simulink model "kf_test"  (R2018b)
settings: Solver=ode2  StartTime=0  StopTime=200  FixedStep=0.002  RelTol=1e-3  EnableMultiTasking=on
model workspace (MAT data in the model file):
  m = 1000
undefined symbols (not defined in the file or in its folder): t_EstimateLoc1_s, t_EstimateLoc2_s, TUMVehicleState
libraries: simulink x6
settings Model: DataDictionary=kf_test.sldd  PauseTimes=42.1  Creator=wischnewski  LastModifiedBy=ge34qer
settings DataIOCC: ExternalInput=input  LoadExternalInput=on  SaveFormat=Structure
settings OptimizationCC: LifeSpan=inf
settings DebuggingCC: MultiTaskRateTransMsg=warning
settings SFSimCC: SimUseLocalCustomCode=off
settings RTWCC: RTWUseLocalCustomCode=off
settings CodeAppCC: StateflowObjectComments=on

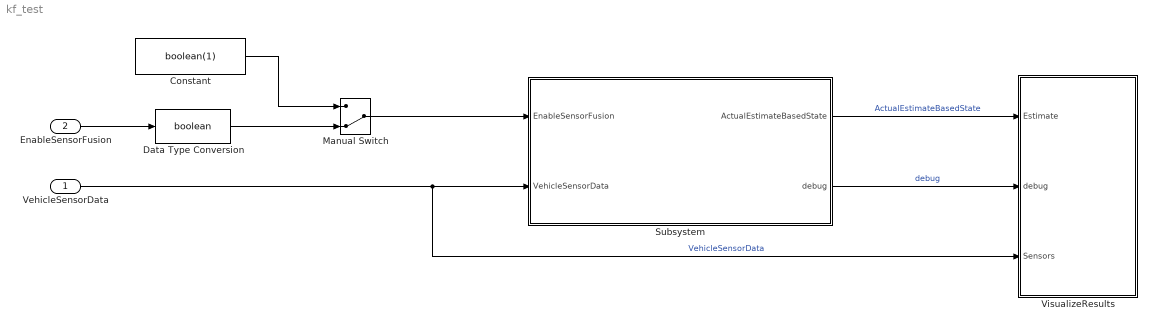
== system kf_test ==
  VehicleSensorData : Inport  OutDataTypeStr=Bus: VehicleSensorData
  EnableSensorFusion : Inport  Port=2  OutDataTypeStr=uint16
  Constant : Constant  Value=boolean(1)
  Data Type Conversion : DataTypeConversion  OutDataTypeStr=boolean
  Manual Switch : ManualSwitch  CurrentSetting=0
  Subsystem : Subsystem
  VisualizeResults : Subsystem
  wires:
  VehicleSensorData/1 -> VisualizeResults/3(Sensors), Subsystem/2(VehicleSensorData)  "VehicleSensorData"
  Subsystem/1(ActualEstimateBasedState) -> VisualizeResults/1(Estimate)  "ActualEstimateBasedState"
  Subsystem/2(debug) -> VisualizeResults/2(debug)  "debug"
  EnableSensorFusion/1 -> Data Type Conversion/1
  Constant/1 -> Manual Switch/1
  Data Type Conversion/1 -> Manual Switch/2
  Manual Switch/1 -> Subsystem/1(EnableSensorFusion)

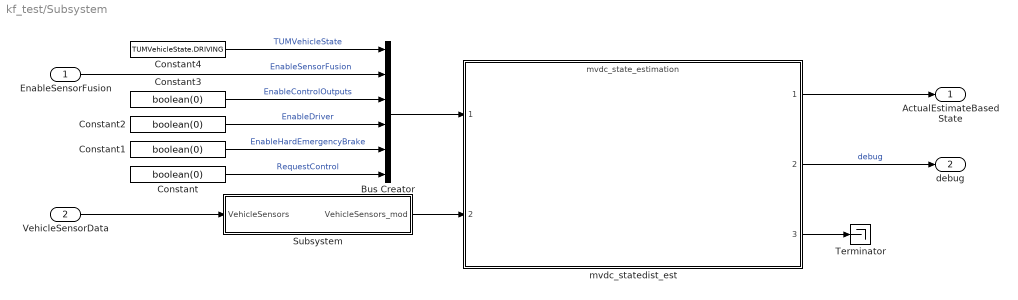
== system kf_test/Subsystem ==
  EnableSensorFusion : Inport
  VehicleSensorData : Inport  Port=2
  Bus Creator : BusCreator  Inputs=6
  Constant{,1..3} (4 alike) : Constant  Value=boolean(0)
  Constant4 : Constant  Value=TUMVehicleState.DRIVING
  Subsystem : Subsystem
  Terminator : Terminator
  mvdc_statedist_est : ModelReference  ModelNameDialog=mvdc_state_estimation  SimulationMode=Normal  ModelReferenceVersion=1.939
  ActualEstimateBasedState : Outport
  debug : Outport  Port=2
  wires:
  mvdc_statedist_est/1 -> ActualEstimateBasedState/1
  mvdc_statedist_est/2 -> debug/1  "debug"
  VehicleSensorData/1 -> Subsystem/1(VehicleSensors)
  Subsystem/1(VehicleSensors_mod) -> mvdc_statedist_est/2
  mvdc_statedist_est/3 -> Terminator/1
  Bus Creator/1 -> mvdc_statedist_est/1
  Constant/1 -> Bus Creator/6  "RequestControl"
  Constant1/1 -> Bus Creator/5  "EnableHardEmergencyBrake"
  Constant2/1 -> Bus Creator/4  "EnableDriver"
  Constant3/1 -> Bus Creator/3  "EnableControlOutputs"
  Constant4/1 -> Bus Creator/1  "TUMVehicleState"
  EnableSensorFusion/1 -> Bus Creator/2  "EnableSensorFusion"

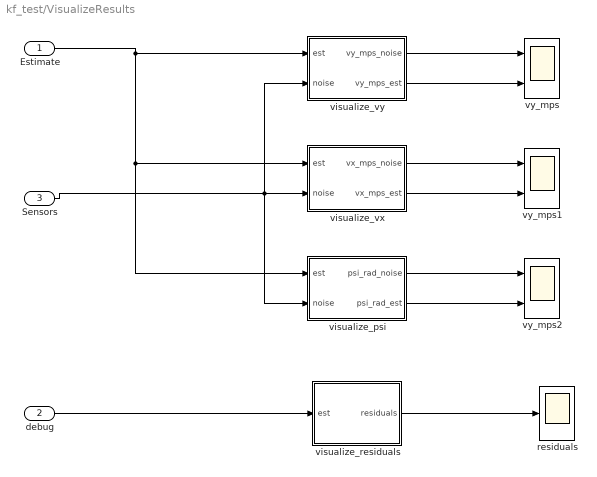
== system kf_test/VisualizeResults ==
  Estimate : Inport
  debug : Inport  Port=2
  Sensors : Inport  Port=3
  residuals : Scope
  visualize_psi : Subsystem
  visualize_residuals : Subsystem
  visualize_vx : Subsystem
  visualize_vy : Subsystem
  vy_mps : Scope  NumInputPorts=2
  vy_mps1 : Scope  NumInputPorts=2
  vy_mps2 : Scope  NumInputPorts=2
  wires:
  visualize_residuals/1(residuals) -> residuals/1
  Estimate/1 -> visualize_psi/1(est), visualize_vx/1(est), visualize_vy/1(est)
  Sensors/1 -> visualize_psi/2(noise), visualize_vy/2(noise), visualize_vx/2(noise)
  debug/1 -> visualize_residuals/1(est)
  visualize_vy/1(vy_mps_noise) -> vy_mps/1
  visualize_vy/2(vy_mps_est) -> vy_mps/2
  visualize_vx/1(vx_mps_noise) -> vy_mps1/1
  visualize_vx/2(vx_mps_est) -> vy_mps1/2
  visualize_psi/1(psi_rad_noise) -> vy_mps2/1
  visualize_psi/2(psi_rad_est) -> vy_mps2/2

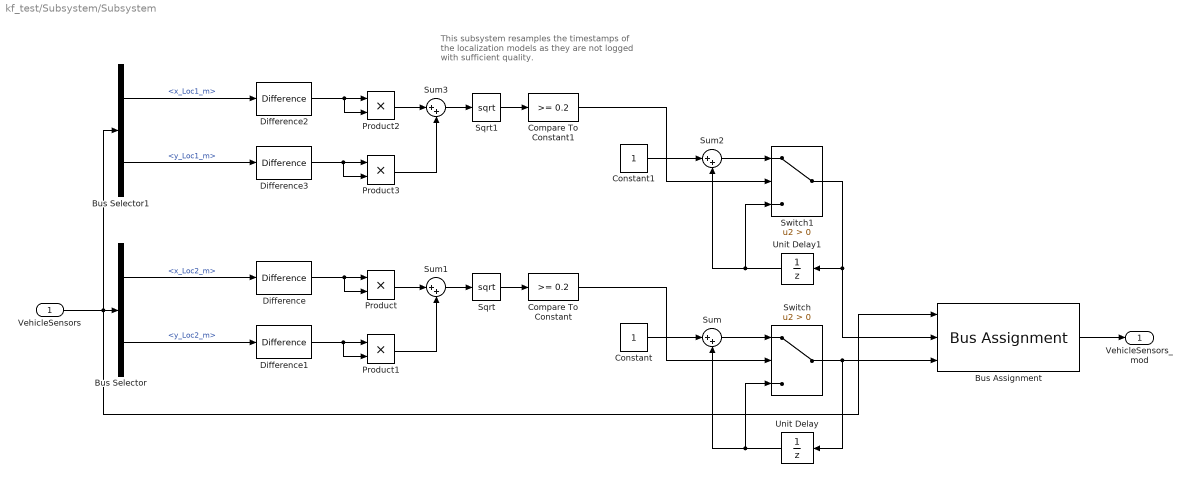
== system kf_test/Subsystem/Subsystem ==
  note: This subsystem resamples the timestamps
      | of the localization models as they are not
      | logged with sufficient quality.
  VehicleSensors : Inport
  Bus Assignment : BusAssignment  AssignedSignals=t_EstimateLoc1_s,t_EstimateLoc2_s
  Bus Selector : BusSelector  OutputSignals=x_Loc2_m,y_Loc2_m
  Bus Selector1 : BusSelector  OutputSignals=x_Loc1_m,y_Loc1_m
  Compare To Constant : simulink/Logic and Bit Operations/Compare To Constant  relop=>=  const=0.2  OutDataTypeStr=boolean
  Compare To Constant1 : simulink/Logic and Bit Operations/Compare To Constant  relop=>=  const=0.2  OutDataTypeStr=boolean
  Constant : Constant
  Constant1 : Constant
  Difference{,1..3} (4 alike) : simulink/Discrete/Difference  ICPrevInput=0.0  OutMin=[]  OutMax=[]  OutDataType=fixdt(1, 16)  OutScaling=2^-10  DoSatur=off
  Product{,1..3} (4 alike) : Product
  Sqrt : Sqrt  SaturateOnIntegerOverflow=on
  Sqrt1 : Sqrt  SaturateOnIntegerOverflow=on
  Sum{,1..3} (4 alike) : Sum  Inputs=|++
  Switch : Switch  Criteria=u2 > Threshold
  Switch1 : Switch  Criteria=u2 > Threshold
  Unit Delay : UnitDelay  SampleTime=-1
  Unit Delay1 : UnitDelay  SampleTime=-1
  VehicleSensors_mod : Outport
  wires:
  Bus Selector/2 -> Difference1/1  "<y_Loc2_m>"
  Unit Delay/1 -> Sum/2, Switch/3
  Difference1/1 -> Product1/2, Product1/1
  Sqrt/1 -> Compare To Constant/1
  Product/1 -> Sum1/1
  Switch/1 -> Unit Delay/1, Bus Assignment/3
  Bus Assignment/1 -> VehicleSensors_mod/1
  Constant/1 -> Sum/1
  Product1/1 -> Sum1/2
  Sum1/1 -> Sqrt/1
  VehicleSensors/1 -> Bus Assignment/1, Bus Selector1/1, Bus Selector/1
  Sum/1 -> Switch/1
  Difference/1 -> Product/2, Product/1
  Bus Selector/1 -> Difference/1  "<x_Loc2_m>"
  Compare To Constant/1 -> Switch/2
  Compare To Constant1/1 -> Switch1/2
  Sqrt1/1 -> Compare To Constant1/1
  Bus Selector1/1 -> Difference2/1  "<x_Loc1_m>"
  Unit Delay1/1 -> Sum2/2, Switch1/3
  Product2/1 -> Sum3/1
  Sum2/1 -> Switch1/1
  Difference3/1 -> Product3/2, Product3/1
  Difference2/1 -> Product2/2, Product2/1
  Switch1/1 -> Bus Assignment/2, Unit Delay1/1
  Bus Selector1/2 -> Difference3/1  "<y_Loc1_m>"
  Constant1/1 -> Sum2/1
  Sum3/1 -> Sqrt1/1
  Product3/1 -> Sum3/2

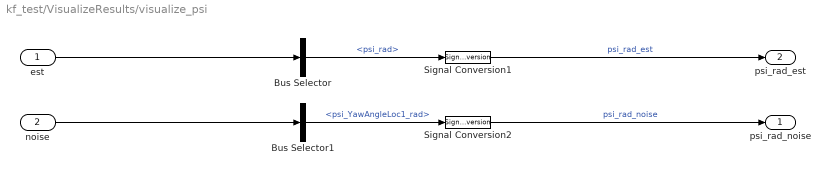
== system kf_test/VisualizeResults/visualize_psi ==
  est : Inport
  noise : Inport  Port=2
  Bus Selector : BusSelector  OutputSignals=Pos.psi_rad
  Bus Selector1 : BusSelector  OutputSignals=psi_YawAngleLoc1_rad
  Signal Conversion1 : SignalConversion  OverrideOpt=off
  Signal Conversion2 : SignalConversion  OverrideOpt=off
  psi_rad_noise : Outport
  psi_rad_est : Outport  Port=2
  wires:
  noise/1 -> Bus Selector1/1
  est/1 -> Bus Selector/1
  Signal Conversion1/1 -> psi_rad_est/1  "psi_rad_est"
  Signal Conversion2/1 -> psi_rad_noise/1  "psi_rad_noise"
  Bus Selector/1 -> Signal Conversion1/1  "<psi_rad>"
  Bus Selector1/1 -> Signal Conversion2/1  "<psi_YawAngleLoc1_rad>"

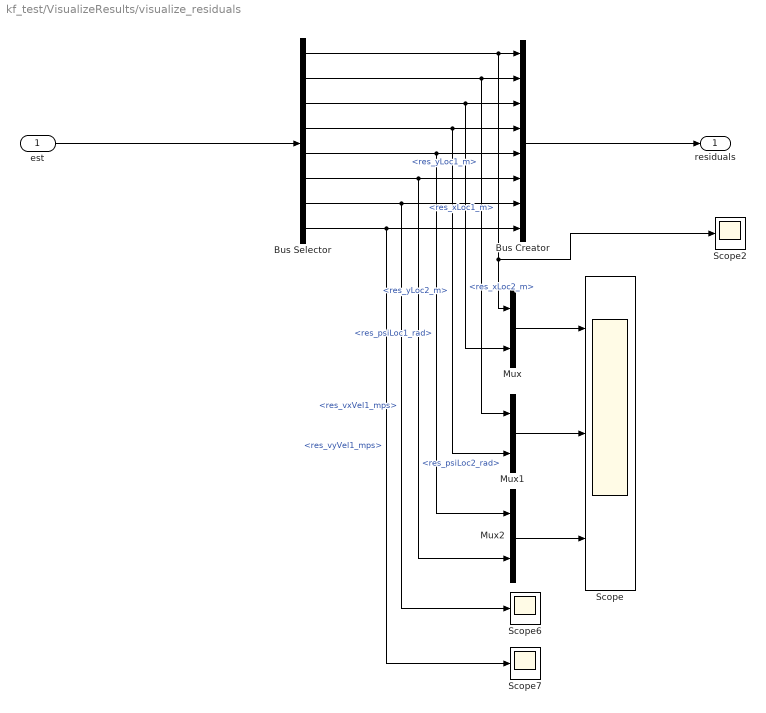
== system kf_test/VisualizeResults/visualize_residuals ==
  est : Inport
  Bus Creator : BusCreator  Inputs=8
  Bus Selector : BusSelector  OutputSignals=Residuals.res_xLoc1_m,Residuals.res_yLoc1_m,Residuals.res_xLoc2_m,Residuals.res_yLoc2_m,Residuals.res_psiLoc1_rad,Residuals.res_psiLoc2_rad,Residuals.res_vxVel1_mps,Residuals.res_vyVel1_mps
  Mux : Mux  Inputs=2
  Mux1 : Mux  Inputs=2
  Mux2 : Mux  Inputs=2
  Scope : Scope  NumInputPorts=3
  Scope2 : Scope
  Scope6 : Scope
  Scope7 : Scope
  residuals : Outport
  wires:
  Bus Selector/1 -> Scope2/1, Mux/1, Bus Creator/1  "<res_xLoc1_m>"
  est/1 -> Bus Selector/1
  Bus Selector/2 -> Mux1/1, Bus Creator/2  "<res_yLoc1_m>"
  Bus Selector/3 -> Mux/2, Bus Creator/3  "<res_xLoc2_m>"
  Bus Selector/5 -> Mux2/1, Bus Creator/5  "<res_psiLoc1_rad>"
  Bus Selector/4 -> Mux1/2, Bus Creator/4  "<res_yLoc2_m>"
  Bus Selector/6 -> Mux2/2, Bus Creator/6  "<res_psiLoc2_rad>"
  Bus Selector/7 -> Scope6/1, Bus Creator/7  "<res_vxVel1_mps>"
  Bus Selector/8 -> Scope7/1, Bus Creator/8  "<res_vyVel1_mps>"
  Bus Creator/1 -> residuals/1
  Mux1/1 -> Scope/2
  Mux/1 -> Scope/1
  Mux2/1 -> Scope/3

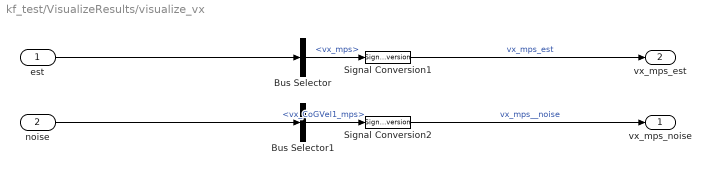
== system kf_test/VisualizeResults/visualize_vx ==
  est : Inport
  noise : Inport  Port=2
  Bus Selector : BusSelector  OutputSignals=vx_mps
  Bus Selector1 : BusSelector  OutputSignals=vx_CoGVel1_mps
  Signal Conversion1 : SignalConversion  OverrideOpt=off
  Signal Conversion2 : SignalConversion  OverrideOpt=off
  vx_mps_noise : Outport
  vx_mps_est : Outport  Port=2
  wires:
  noise/1 -> Bus Selector1/1
  est/1 -> Bus Selector/1
  Signal Conversion1/1 -> vx_mps_est/1  "vx_mps_est"
  Signal Conversion2/1 -> vx_mps_noise/1  "vx_mps__noise"
  Bus Selector/1 -> Signal Conversion1/1  "<vx_mps>"
  Bus Selector1/1 -> Signal Conversion2/1  "<vx_CoGVel1_mps>"

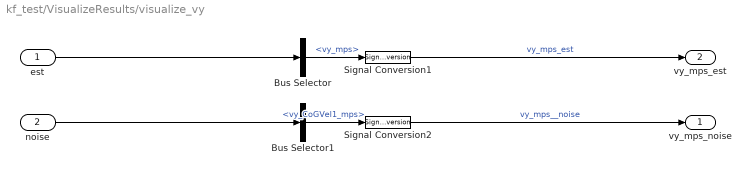
== system kf_test/VisualizeResults/visualize_vy ==
  est : Inport
  noise : Inport  Port=2
  Bus Selector : BusSelector  OutputSignals=vy_mps
  Bus Selector1 : BusSelector  OutputSignals=vy_CoGVel1_mps
  Signal Conversion1 : SignalConversion  OverrideOpt=off
  Signal Conversion2 : SignalConversion  OverrideOpt=off
  vy_mps_noise : Outport
  vy_mps_est : Outport  Port=2
  wires:
  Bus Selector1/1 -> Signal Conversion2/1  "<vy_CoGVel1_mps>"
  Bus Selector/1 -> Signal Conversion1/1  "<vy_mps>"
  Signal Conversion2/1 -> vy_mps_noise/1  "vy_mps__noise"
  Signal Conversion1/1 -> vy_mps_est/1  "vy_mps_est"
  est/1 -> Bus Selector/1
  noise/1 -> Bus Selector1/1
